simulink model "Encoder_reader_simulink"  (R2025a)
settings: Solver=FixedStepAuto  StartTime=0.0  StopTime=inf  FixedStep=0.001  RelTol=1e-3  EnableMultiTasking=on
libraries: stm32g4xxblockslib x3, stm32f4xxblockslib x2
settings Model: STM32="{\"EncoderBlockForG4\":[{\"ID\":\"untitled:1\"},{\"ID\":\"Lab3_Encoder:1\"},{\"ID\":\"Encoder_reader_simulink:1\"},{\"ID\":\"Encoder_reader_simulink:23\"},{\"ID\":\"Encoder_reader_simulink:24\"}],\"DigitalPortRead\":[{\"ID\":\"Encoder_reader_simulink:20\"},{\"ID\":\"Encoder_reader_simulink:21\"}]}"  Creator=User  LastModifiedBy=Yhommy's Notebook
settings OptimizationCC: DefaultParameterBehavior=Inlined  EnhancedBackFolding=on  PassReuseOutputArgsAs=Individual arguments  ZeroExternalMemoryAtStartup=off  ZeroInternalMemoryAtStartup=off  MaxStackSize=512  OptimizeBlockOrder=speed  DifferentSizesBufferReuse=on  OptimizationCustomize=off  EfficientTunableParamExpr=on
settings DebuggingCC: ParameterTunabilityLossMsg=error
settings HardwareCC: ProdBitPerPointer=32.0  ProdBitPerSizeT=32.0  ProdBitPerPtrDiffT=32.0  ProdLargestAtomicInteger=Long  ProdLargestAtomicFloat=Double  ProdWordSize=32.0  ProdLongLongMode=on  ProdHWDeviceType=ARM Compatible->ARM Cortex-M
settings SFSimCC: MATLABDynamicMemAlloc=off
settings RTWCC: SystemTargetFile=ert.tlc  HardwareBoard=STM32G4xx Based  TemplateMakefile=ert_default_tmf  Toolchain=GNU Tools for ARM Embedded Processors  Description=Embedded Coder
settings CodeAppCC: ForceParamTrailComments=on  IgnoreCustomStorageClasses=off  OperatorAnnotations=on  SimulinkDataObjDesc=on  SFDataObjDesc=on  InsertBlockDesc=on
settings ERTTargetCC: ExtModeTransport=3.0  ExtModeStaticAllocSize=2048.0  TargetLangStandard=C99 (ISO)  CodeReplacementLibrary=ARM Cortex-M  SupportContinuousTime=on

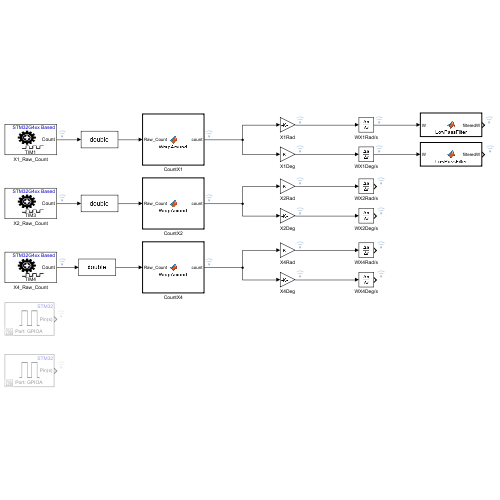
[thumbnail: Simulink's stored preview of the top-level diagram]
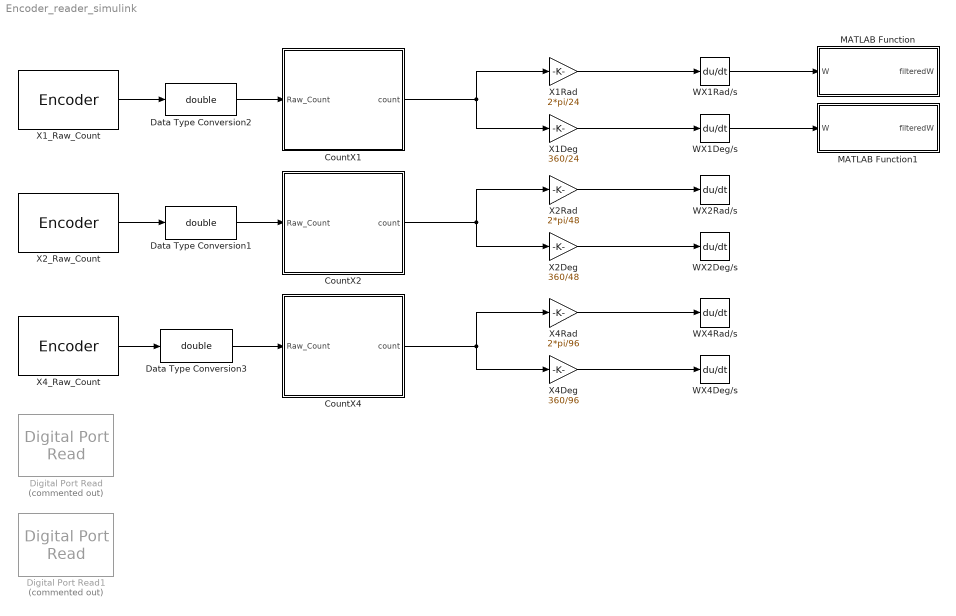
== system Encoder_reader_simulink ==
  CountX1 : MATLAB Function  TreatAsAtomicUnit=on
  CountX2 : MATLAB Function  TreatAsAtomicUnit=on
  CountX4 : MATLAB Function  TreatAsAtomicUnit=on
  Data Type Conversion1 : DataTypeConversion  OutDataTypeStr=double  SaturateOnIntegerOverflow=off  RndMeth=Floor
  Data Type Conversion2 : DataTypeConversion  OutDataTypeStr=double  SaturateOnIntegerOverflow=off  RndMeth=Floor
  Data Type Conversion3 : DataTypeConversion  OutDataTypeStr=double  SaturateOnIntegerOverflow=off  RndMeth=Floor
  Digital Port Read : stm32f4xxblockslib/Digital Port Read  Commented=on  PortName=GPIOA  PinNumber=4  ReadOperation=on  IOAsArray=on  SampleTime=-1  EnableSimPort=off  hoistedMaskSrc=ECSoC/ECSimCodegen/Digital Port Read
  Digital Port Read1 : stm32f4xxblockslib/Digital Port Read  Commented=on  PortName=GPIOA  PinNumber=6  ReadOperation=on  IOAsArray=on  SampleTime=-1  EnableSimPort=off  hoistedMaskSrc=ECSoC/ECSimCodegen/Digital Port Read
  MATLAB Function : MATLAB Function  TreatAsAtomicUnit=on
  MATLAB Function1 : MATLAB Function  TreatAsAtomicUnit=on
  WX1Deg/s : Derivative
  WX1Rad/s : Derivative
  WX2Deg/s : Derivative
  WX2Rad/s : Derivative
  WX4Deg/s : Derivative
  WX4Rad/s : Derivative
  X1Deg : Gain  Gain=360/24
  X1Rad : Gain  Gain=2*pi/24
  X1_Raw_Count : stm32g4xxblockslib/Encoder  TimerModule=TIM1  EnableResetInput=off  OutputCountAfterFirstIndex=off  OutputValidIndex=off  OutputDirection=off  OutputStatus=off  SampleTime=-1
  X2Deg : Gain  Gain=360/48
  X2Rad : Gain  Gain=2*pi/48
  X2_Raw_Count : stm32g4xxblockslib/Encoder  TimerModule=TIM3  EnableResetInput=off  OutputCountAfterFirstIndex=off  OutputValidIndex=off  OutputDirection=off  OutputStatus=off  SampleTime=-1
  X4Deg : Gain  Gain=360/96
  X4Rad : Gain  Gain=2*pi/96
  X4_Raw_Count : stm32g4xxblockslib/Encoder  TimerModule=TIM4  EnableResetInput=off  OutputCountAfterFirstIndex=off  OutputValidIndex=off  OutputDirection=off  OutputStatus=off  SampleTime=-1
  wires:
  X2_Raw_Count/1 -> Data Type Conversion1/1
  Data Type Conversion1/1 -> CountX2/1(Raw_Count)
  X1_Raw_Count/1 -> Data Type Conversion2/1
  X4_Raw_Count/1 -> Data Type Conversion3/1
  Data Type Conversion2/1 -> CountX1/1(Raw_Count)
  Data Type Conversion3/1 -> CountX4/1(Raw_Count)
  X1Rad/1 -> WX1Rad/s/1
  X1Deg/1 -> WX1Deg/s/1
  X4Deg/1 -> WX4Deg/s/1
  X4Rad/1 -> WX4Rad/s/1
  X2Deg/1 -> WX2Deg/s/1
  X2Rad/1 -> WX2Rad/s/1
  CountX1/1(count) -> X1Deg/1, X1Rad/1
  CountX2/1(count) -> X2Deg/1, X2Rad/1
  CountX4/1(count) -> X4Rad/1, X4Deg/1
  WX1Rad/s/1 -> MATLAB Function/1(W)
  WX1Deg/s/1 -> MATLAB Function1/1(W)

== matlab function Encoder_reader_simulink/CountX2 ==
  data: Raw_Count input; count output
function count = WrapAround(Raw_Count)
    persistent current_count
    persistent last_count

    if isempty(current_count)
        current_count = 0;
    end
    if isempty(last_count)
        last_count = Raw_Count;
    end

    delta_count = Raw_Count - last_count;

    if delta_count >= 61439
        current_count = current_count - 1;
    elseif delta_count <= -61439
        current_count = current_count + 1;
    else
        current_count = current_count + delta_count;
    end

    last_count = Raw_Count;

    count = current_count;
end

== matlab function Encoder_reader_simulink/CountX4 ==
  data: Raw_Count input; count output
function count = WrapAround(Raw_Count)
    persistent current_count
    persistent last_count

    if isempty(current_count)
        current_count = 0;
    end
    if isempty(last_count)
        last_count = Raw_Count;
    end

    delta_count = Raw_Count - last_count;

    if delta_count >= 61439
        current_count = current_count - 1;
    elseif delta_count <= -61439
        current_count = current_count + 1;
    else
        current_count = current_count + delta_count;
    end

    last_count = Raw_Count;

    count = current_count;
end

== matlab function Encoder_reader_simulink/MATLAB Function ==
  data: W input; filteredW output
function filteredW = LowPassFilter(W)

    persistent prevFiltered prevW

    if isempty(prevFiltered)
        prevFiltered = 0;
    end
    if isempty(prevW)
        prevW = 0;
    end

    filteredW = 0.96906992 * prevFiltered + ...
                0.01546504 * W + ...
                0.01546504 * prevW;

    prevFiltered = filteredW;
    prevW = W;
end

== matlab function Encoder_reader_simulink/MATLAB Function1 ==
  data: W input; filteredW output
function filteredW = LowPassFilter(W)

    persistent prevFiltered prevW

    if isempty(prevFiltered)
        prevFiltered = 0;
    end
    if isempty(prevW)
        prevW = 0;
    end

    filteredW = 0.96906992 * prevFiltered + ...
                0.01546504 * W + ...
                0.01546504 * prevW;

    prevFiltered = filteredW;
    prevW = W;
end

== matlab function Encoder_reader_simulink/CountX1 ==
  data: Raw_Count input; count output
function count = WrapAround(Raw_Count)
    persistent current_count
    persistent last_count

    if isempty(current_count)
        current_count = 0;
    end
    if isempty(last_count)
        last_count = Raw_Count;
    end

    delta_count = Raw_Count - last_count;

    if delta_count >= 61439
        current_count = current_count - 1;
    elseif delta_count <= -61439
        current_count = current_count + 1;
    else
        current_count = current_count + delta_count;
    end

    last_count = Raw_Count;

    count = current_count;
end
